simulink library "lib_Controller"  (R2017a)
settings: Solver=VariableStepAuto  StartTime=0.0  StopTime=10.0  RelTol=1e-3
undefined symbols (not defined in the file): cal, eng, ENGTRQ_MSMCH_Degraded_CP, ENGTRQ_MSMCH_ErrCritical_CP, ENGTRQ_MSMCH_LimpHome_CP
libraries: simulink x58, powerlib_meascontrol x3, lib_SystemDiag x1, EC2_libraries x1, lib_FuelManager x1, lib_TorqueDistribution x1
(part 3 of 3)

== system lib_Controller/Controller_with_Transmission_Manager1/HSC/Camaro Fault Detection/Signal Diagnostic/ESS Signal Diagnostic/Max charging voltage fault detect ==
  note: Note: When the ESS receives the energy from grid or regenerative braking,
      | the charging voltage to the inverter can not be bigger than 419V, otherwise the MCU will set to fault
  In1 : Inport
  " " : simulink/Logic and Bit Operations/Compare To Constant  relop=>  const=419  OutDataTypeStr=boolean
  Abs : Abs
  Compare To Zero : simulink/Logic and Bit Operations/Compare To Zero  relop=<  OutDataTypeStr=boolean
  Logical Operator : Logic  AllPortsSameDT=off  OutDataTypeStr=boolean
  Out1 : Outport
  wires:
  Abs/1 -> " "/1
  Logical Operator/1 -> Out1/1
  " "/1 -> Logical Operator/1
  In1/1 -> Compare To Zero/1, Abs/1
  Compare To Zero/1 -> Logical Operator/2

== system lib_Controller/Controller_with_Transmission_Manager1/HSC/Camaro Fault Detection/Signal Diagnostic/ESS Signal Diagnostic/Rolling Alive Counter Detection ==
  In1 : Inport
  Chart : Stateflow chart  TreatAsAtomicUnit=on
  Constant : Constant  Value=0.01
  Constant1 : Constant  Value=0.01
  Detect Change : simulink/Logic and Bit Operations/Detect Change  vinit=1  InputProcessing=Inherited  OutDataTypeStr=boolean
  Out1 : Outport
  wires:
  Constant1/1 -> Chart/3(tloop)
  In1/1 -> Detect Change/1
  Detect Change/1 -> Chart/1(PulseDetect)
  Chart/1(flag) -> Out1/1
  Constant/1 -> Chart/2(CycleTime)

== system lib_Controller/Controller_with_Transmission_Manager1/HSC/Camaro Fault Detection/Signal Diagnostic/ESS Signal Diagnostic/Validity Check ==
  In1 : Inport
  " Normal Operation" : simulink/Logic and Bit Operations/Compare To Constant  relop===  const=1  OutDataTypeStr=boolean
  Below Normal Operation : simulink/Logic and Bit Operations/Compare To Constant  relop===  const=0  OutDataTypeStr=boolean
  Logical Operator : Logic  Operator=OR  AllPortsSameDT=off  OutDataTypeStr=boolean
  Out1 : Outport
  wires:
  In1/1 -> Below Normal Operation/1, " Normal Operation"/1
  Below Normal Operation/1 -> Logical Operator/1
  " Normal Operation"/1 -> Logical Operator/2
  Logical Operator/1 -> Out1/1  "BMSgdf_SigValid"

== system lib_Controller/Controller_with_Transmission_Manager1/HSC/Camaro Fault Detection/Signal Diagnostic/Engine Signal Diagnostic/EngTempValidity_Check ==
  In1 : Inport
  Above Normal Operation : simulink/Logic and Bit Operations/Compare To Constant  relop===  const=3  OutDataTypeStr=boolean
  Logical Operator1 : Logic  Operator=NOT  AllPortsSameDT=off  OutDataTypeStr=boolean
  Out1 : Outport
  wires:
  Logical Operator1/1 -> Out1/1
  Above Normal Operation/1 -> Logical Operator1/1
  In1/1 -> Above Normal Operation/1

== system lib_Controller/Controller_with_Transmission_Manager1/HSC/Camaro Fault Detection/Signal Diagnostic/Engine Signal Diagnostic/Rolling Alive Counter Detection1 ==
  In1 : Inport
  Chart : Stateflow chart  TreatAsAtomicUnit=on
  Constant : Constant  Value=0.01
  Detect Change : simulink/Logic and Bit Operations/Detect Change  vinit=1  InputProcessing=Inherited  OutDataTypeStr=boolean
  Out1 : Outport
  wires:
  Constant/1 -> Chart/2(CycleTime)
  Chart/1(flag) -> Out1/1
  Detect Change/1 -> Chart/1(PulseDetect)
  In1/1 -> Detect Change/1

== system lib_Controller/Controller_with_Transmission_Manager1/HSC/Camaro Fault Detection/Signal Diagnostic/Transmission Signal Diagnostic/Rolling Alive Counter Detection ==
  In1 : Inport
  Chart : Stateflow chart  TreatAsAtomicUnit=on
  Constant : Constant  Value=0.01
  Detect Change : simulink/Logic and Bit Operations/Detect Change  vinit=1  InputProcessing=Inherited  OutDataTypeStr=boolean
  Out1 : Outport
  wires:
  Constant/1 -> Chart/2(CycleTime)
  Chart/1(flag) -> Out1/1
  Detect Change/1 -> Chart/1(PulseDetect)
  In1/1 -> Detect Change/1

== system lib_Controller/Controller_with_Transmission_Manager1/HSC/Camaro Fault Detection/Signal Diagnostic/Transmission Signal Diagnostic/Vehicle Direction Fault Detection ==
  LvrPosTrnsShft : Inport
  Speed : Inport  Port=2
  Compare To Constant : simulink/Logic and Bit Operations/Compare To Constant  relop===  const=4  OutDataTypeStr=boolean
  Compare To Constant1 : simulink/Logic and Bit Operations/Compare To Constant  relop=<  const=0  OutDataTypeStr=boolean
  Compare To Constant2 : simulink/Logic and Bit Operations/Compare To Constant  relop===  const=2  OutDataTypeStr=boolean
  Compare To Constant3 : simulink/Logic and Bit Operations/Compare To Constant  relop=>  const=0  OutDataTypeStr=boolean
  Logical Operator : Logic  AllPortsSameDT=off  OutDataTypeStr=boolean
  Logical Operator1 : Logic  AllPortsSameDT=off  OutDataTypeStr=boolean
  Logical Operator2 : Logic  Operator=OR  AllPortsSameDT=off  OutDataTypeStr=boolean
  Out1 : Outport
  wires:
  Logical Operator2/1 -> Out1/1
  Logical Operator/1 -> Logical Operator2/2
  Logical Operator1/1 -> Logical Operator2/1
  Compare To Constant3/1 -> Logical Operator1/2
  Compare To Constant2/1 -> Logical Operator1/1
  Compare To Constant/1 -> Logical Operator/1
  Compare To Constant1/1 -> Logical Operator/2
  Speed/1 -> Compare To Constant1/1, Compare To Constant3/1
  LvrPosTrnsShft/1 -> Compare To Constant/1, Compare To Constant2/1

== system lib_Controller/Controller_with_Transmission_Manager1/HSC/Driver_Requests/APP_BPP to DrvIntndAxlTrq2/Post Driver Intnded Axle Torque/Brake Command ==
  APP : Inport
  BPP : Inport  Port=2
  VehicleSpeed : Inport  Port=3
  1-D Lookup Table : Lookup_n-D  NumberOfTableDimensions=1  BreakpointsForDimension1=cal.Regen.BrakeAxleTrq.idx1_BrkPdlPos  Table=cal.Regen.BrakeAxleTrq.map  InternalRulePriority=Speed  RndMeth=Simplest  InputSameDT=on
  Compare To Constant : simulink/Logic and Bit Operations/Compare To Constant  relop=>=  const=cal.Regen.EnableSpeed  OutDataTypeStr=boolean
  Compare To Constant4 : simulink/Logic and Bit Operations/Compare To Constant  relop=<=  const=cal.Regen.EnableAPP  OutDataTypeStr=boolean
  Compare To Constant5 : simulink/Logic and Bit Operations/Compare To Constant  relop=>=  const=cal.Regen.DisableAPP  OutDataTypeStr=boolean
  Constant5 : Constant  Value=0
  Latch : Subsystem
  RegenCal : Gain  Gain=1.3
  Switch : Switch  Criteria=u2 > Threshold
  Terminator : Terminator
  BrkAxlTrq : Outport
  wires:
  VehicleSpeed/1 -> Compare To Constant/1
  1-D Lookup Table/1 -> RegenCal/1
  Switch/1 -> BrkAxlTrq/1
  APP/1 -> Compare To Constant5/1, Compare To Constant4/1
  BPP/1 -> 1-D Lookup Table/1
  Compare To Constant/1 -> Switch/2
  Constant5/1 -> Switch/3
  Compare To Constant5/1 -> Latch/2(Reset)
  Compare To Constant4/1 -> Latch/1(Input)
  Latch/1(Out1) -> Terminator/1
  RegenCal/1 -> Switch/1

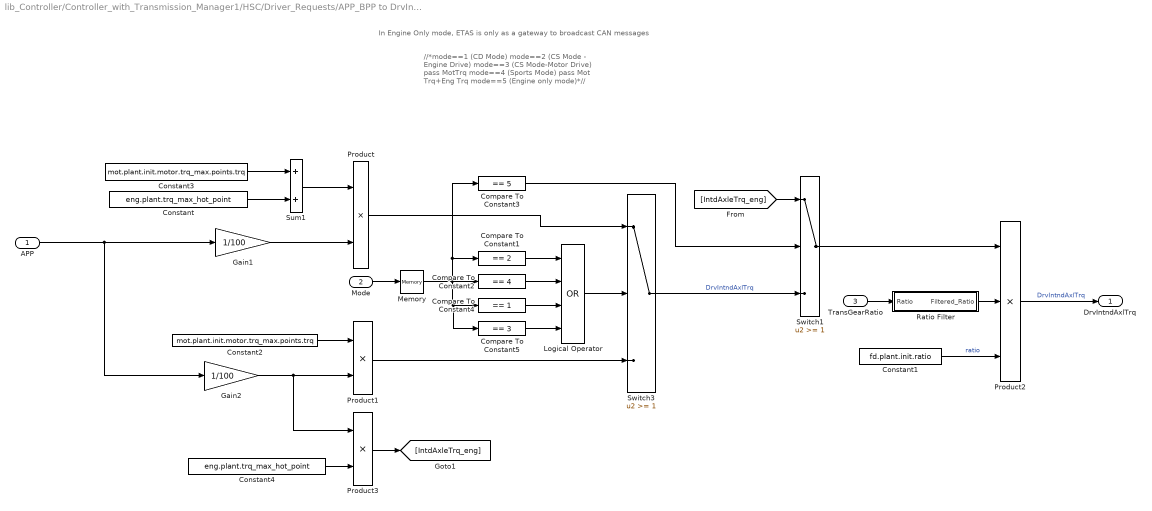
== system lib_Controller/Controller_with_Transmission_Manager1/HSC/Driver_Requests/APP_BPP to DrvIntndAxlTrq2/Post Driver Intnded Axle Torque/Driver Intended Axle Torque ==
  note: In Engine Only mode, ETAS is only as a gateway to broadcast CAN messages
  note: //*mode==1 (CD Mode)
      | mode==2 (CS Mode - Engine Drive)
      | mode==3 (CS Mode-Motor Drive) pass MotTrq
      | mode==4 (Sports Mode) pass Mot Trq+Eng Trq
      | mode==5 (Engine only mode)*//
  APP : Inport
  Mode : Inport  Port=2
  TransGearRatio : Inport  Port=3
  Compare To Constant1 : simulink/Logic and Bit Operations/Compare To Constant  relop===  const=2  OutDataTypeStr=boolean
  Compare To Constant2 : simulink/Logic and Bit Operations/Compare To Constant  relop===  const=4  OutDataTypeStr=boolean
  Compare To Constant3 : simulink/Logic and Bit Operations/Compare To Constant  relop===  const=5  OutDataTypeStr=boolean
  Compare To Constant4 : simulink/Logic and Bit Operations/Compare To Constant  relop===  const=1  OutDataTypeStr=boolean
  Compare To Constant5 : simulink/Logic and Bit Operations/Compare To Constant  relop===  const=3  OutDataTypeStr=boolean
  Constant : Constant  Value=eng.plant.trq_max_hot_point  VectorParams1D=off
  Constant1 : Constant  Value=fd.plant.init.ratio
  Constant2 : Constant  Value=mot.plant.init.motor.trq_max.points.trq  VectorParams1D=off
  Constant3 : Constant  Value=mot.plant.init.motor.trq_max.points.trq  VectorParams1D=off
  Constant4 : Constant  Value=eng.plant.trq_max_hot_point  VectorParams1D=off
  Gain1 : Gain  Gain=1/100
  Gain2 : Gain  Gain=1/100
  Logical Operator : Logic  Operator=OR  Inputs=4  AllPortsSameDT=off  OutDataTypeStr=boolean
  Memory : Memory
  Product : Product  RndMeth=Zero
  Product1 : Product  RndMeth=Zero
  Product2 : Product  Inputs=3  RndMeth=Zero
  Product3 : Product  RndMeth=Zero
  Ratio Filter : Subsystem
  Sum1 : Sum
  Switch1 : Switch  Threshold=1
  Switch3 : Switch  Threshold=1
  DrvIntndAxlTrq : Outport
  wires:
  Constant2/1 -> Product1/1
  Ratio Filter/1(Filtered_Ratio) -> Product2/2
  Gain2/1 -> Product1/2, Product3/1
  Product/1 -> Switch3/1
  Mode/1 -> Memory/1
  Constant1/1 -> Product2/3  "ratio"
  Product1/1 -> Switch3/3
  TransGearRatio/1 -> Ratio Filter/1(Ratio)
  Product2/1 -> DrvIntndAxlTrq/1  "DrvIntndAxlTrq"
  Gain1/1 -> Product/2
  Memory/1 -> Compare To Constant5/1, Compare To Constant4/1, Compare To Constant2/1, Compare To Constant3/1, Compare To Constant1/1
  Constant3/1 -> Sum1/1
  Compare To Constant1/1 -> Logical Operator/1
  Sum1/1 -> Product/1
  Compare To Constant2/1 -> Logical Operator/2
  Constant/1 -> Sum1/2
  Switch3/1 -> Switch1/3  "DrvIntndAxlTrq"
  Product3/1 -> [IntdAxleTrq_eng]
  Compare To Constant3/1 -> Switch1/2
  Constant4/1 -> Product3/2
  Logical Operator/1 -> Switch3/2
  [IntdAxleTrq_eng] -> Switch1/1
  Switch1/1 -> Product2/1
  APP/1 -> Gain2/1, Gain1/1
  Compare To Constant4/1 -> Logical Operator/3
  Compare To Constant5/1 -> Logical Operator/4

== system lib_Controller/Controller_with_Transmission_Manager1/HSC/Powertrain Manager/HV Manager/BMS_Manager/Fault Latch ==
  IsoFault : Inport
  Off Delay : powerlib_meascontrol/Logic/On Delay  DelayType=Off delay  delay=3  ic=0  Ts=0
      settings: SourceProductName=Simscape Power Systems
  IsoFaultLatched : Outport
  wires:
  IsoFault/1 -> Off Delay/1
  Off Delay/1 -> IsoFaultLatched/1

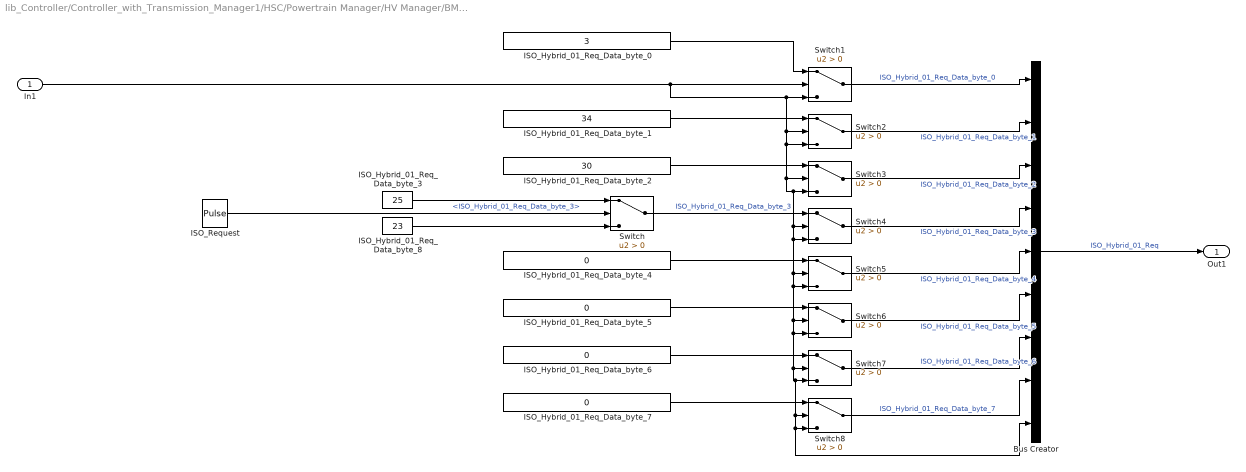
== system lib_Controller/Controller_with_Transmission_Manager1/HSC/Powertrain Manager/HV Manager/BMS_Manager/ISO_Hybrid_01_Req ==
  In1 : Inport
  Bus Creator : BusCreator  Inputs=9
  ISO_Hybrid_01_Req_Data_byte_0 : Constant  Value=3
  ISO_Hybrid_01_Req_Data_byte_1 : Constant  Value=34
  ISO_Hybrid_01_Req_Data_byte_2 : Constant  Value=30
  ISO_Hybrid_01_Req_Data_byte_3 : Constant  Value=25
  ISO_Hybrid_01_Req_Data_byte_{4..7} (4 alike) : Constant  Value=0
  ISO_Hybrid_01_Req_Data_byte_8 : Constant  Value=23
  ISO_Request : DiscretePulseGenerator  PulseType=Time based  Period=0.5  PulseWidth=50  SampleTime=-1
  Switch{,1..8} (9 alike) : Switch  Criteria=u2 > Threshold
  Out1 : Outport
  wires:
  Bus Creator/1 -> Out1/1  "ISO_Hybrid_01_Req"
  Switch6/1 -> Bus Creator/6  "ISO_Hybrid_01_Req_Data_byte_5"
  ISO_Hybrid_01_Req_Data_byte_8/1 -> Switch/3
  Switch5/1 -> Bus Creator/5  "ISO_Hybrid_01_Req_Data_byte_4"
  Switch3/1 -> Bus Creator/3  "ISO_Hybrid_01_Req_Data_byte_2"
  ISO_Hybrid_01_Req_Data_byte_3/1 -> Switch/1
  Switch1/1 -> Bus Creator/1  "ISO_Hybrid_01_Req_Data_byte_0"
  Switch7/1 -> Bus Creator/7  "ISO_Hybrid_01_Req_Data_byte_6"
  Switch2/1 -> Bus Creator/2  "ISO_Hybrid_01_Req_Data_byte_1"
  Switch8/1 -> Bus Creator/8  "ISO_Hybrid_01_Req_Data_byte_7"
  Switch4/1 -> Bus Creator/4  "ISO_Hybrid_01_Req_Data_byte_3"
  ISO_Hybrid_01_Req_Data_byte_0/1 -> Switch1/1
  In1/1 -> Switch2/2, Switch3/3, Switch4/3, Switch5/3, Switch6/3, Switch7/2, Switch7/3, Switch8/2, Bus Creator/9, Switch8/3, Switch6/2, Switch5/2, Switch4/2, Switch3/2, Switch2/3, Switch1/3, Switch1/2
  ISO_Hybrid_01_Req_Data_byte_1/1 -> Switch2/1
  ISO_Hybrid_01_Req_Data_byte_2/1 -> Switch3/1
  Switch/1 -> Switch4/1  "ISO_Hybrid_01_Req_Data_byte_3"
  ISO_Hybrid_01_Req_Data_byte_4/1 -> Switch5/1
  ISO_Hybrid_01_Req_Data_byte_5/1 -> Switch6/1
  ISO_Hybrid_01_Req_Data_byte_6/1 -> Switch7/1
  ISO_Hybrid_01_Req_Data_byte_7/1 -> Switch8/1
  ISO_Request/1 -> Switch/2  "<ISO_Hybrid_01_Req_Data_byte_3>"

== system lib_Controller/Controller_with_Transmission_Manager1/HSC/Powertrain Manager/HV Manager/BMS_Manager/Isolation Fault Calculation ==
  note: This block  allows to know which HV main
      | is having issues. HV POS 25, HV NEG 23.
  Sensors1 : Inport
  Bus Selector5 : BusSelector  OutputSignals=from_CAN.fromEBCAN.from_BMSAntrieb.ISO_Hybrid_01_Resp_Data.ISO_Hybrid_01_Resp_Data_byte_3,from_CAN.fromEBCAN.from_BMSAntrieb.ISO_Hybrid_01_Resp_Data.ISO_Hybrid_01_Resp_Data_byte_4,from_CAN.fromEBCAN.from_BMSAntrieb.ISO_Hybrid_01_Resp_Data.ISO_Hybrid_01_Resp_Data_byte_5
  Compare To Constant : simulink/Logic and Bit Operations/Compare To Constant  relop===  const=23  OutDataTypeStr=boolean
  Compare To Constant1 : simulink/Logic and Bit Operations/Compare To Constant  relop===  const=25  OutDataTypeStr=boolean
  HVnegativeISO : Constant  Value=0
  HVpositiveISO : Constant
  Logical Operator : Logic  Operator=OR  AllPortsSameDT=off  OutDataTypeStr=boolean
  POS or NEG HV MAIN : Switch  Criteria=u2 > Threshold  Threshold=24
  Resistance_Measurement : Subsystem
  Terminator8 : Terminator
  IsoFault : Outport
  wires:
  Resistance_Measurement/1(IsoFault) -> IsoFault/1
  POS or NEG HV MAIN/1 -> Terminator8/1
  Bus Selector5/2 -> Resistance_Measurement/1(In1)  "<ISO_Hybrid_01_Resp_Data_byte_4>"
  Bus Selector5/3 -> Resistance_Measurement/2(In2)  "<ISO_Hybrid_01_Resp_Data_byte_5>"
  Sensors1/1 -> Bus Selector5/1
  HVpositiveISO/1 -> POS or NEG HV MAIN/1
  Bus Selector5/1 -> POS or NEG HV MAIN/2, Compare To Constant1/1, Compare To Constant/1  "<ISO_Hybrid_01_Resp_Data_byte_3>"
  HVnegativeISO/1 -> POS or NEG HV MAIN/3
  Compare To Constant1/1 -> Logical Operator/1
  Compare To Constant/1 -> Logical Operator/2
  Logical Operator/1 -> Resistance_Measurement/Enable

== system lib_Controller/Controller_with_Transmission_Manager1/HSC/Powertrain Manager/HV Manager/DCDC Manager/Contactors status check ==
  note: Note: Contactors don't close when commanded
  BMS_Voltage : Inport
  BMS_LinkVoltage : Inport  Port=2
  BMS_HVILfault : Inport  Port=3
  " " : simulink/Logic and Bit Operations/Compare To Constant  relop=>  const=2  OutDataTypeStr=boolean
  Abs : Abs
  Logical Operator : Logic  Operator=OR  AllPortsSameDT=off  OutDataTypeStr=boolean
  Sum : Sum  Inputs=+-
  Out1 : Outport
  wires:
  BMS_Voltage/1 -> Sum/1
  Logical Operator/1 -> Out1/1  "BMS_contactorsFailed_Detected"
  Sum/1 -> Abs/1
  Abs/1 -> " "/1
  BMS_LinkVoltage/1 -> Sum/2
  BMS_HVILfault/1 -> Logical Operator/2
  " "/1 -> Logical Operator/1  "BMS_contactorsFailed_SigValid"

== system lib_Controller/Controller_with_Transmission_Manager1/HSC/Powertrain Manager/HV Manager/DCDC Manager/DCModeOverride ==
  In1 : Inport
  DCDCOVrrdSwitch : Constant  Value=0
  DCDCOVrrdVal : Constant  Value=0
  Switch : Switch  Criteria=u2 > Threshold
  Out1 : Outport
  wires:
  Switch/1 -> Out1/1  "DC_mode"
  In1/1 -> Switch/3
  DCDCOVrrdSwitch/1 -> Switch/2
  DCDCOVrrdVal/1 -> Switch/1

== system lib_Controller/Controller_with_Transmission_Manager1/HSC/Powertrain Manager/HV Manager/Inverter Manager/RequestOverride ==
  In1 : Inport
  ReqStateOVrRDSwitch : Constant  Value=0
  RequestedStateOvrRdValue : Constant
  Switch : Switch  Criteria=u2 > Threshold
  Out1 : Outport
  wires:
  Switch/1 -> Out1/1  "VCU_RequestedStateINV"
  In1/1 -> Switch/3
  ReqStateOVrRDSwitch/1 -> Switch/2
  RequestedStateOvrRdValue/1 -> Switch/1

== system lib_Controller/Controller_with_Transmission_Manager1/HSC/Camaro Fault Detection/Signal Diagnostic/ESS Signal Diagnostic/ESS SOC Validity Check/essSOCValidity_Check ==
  In1 : Inport
  Above Normal Operation : simulink/Logic and Bit Operations/Compare To Constant  relop===  const=3  OutDataTypeStr=boolean
  Below Normal Operation : simulink/Logic and Bit Operations/Compare To Constant  relop===  const=0  OutDataTypeStr=boolean
  Logical Operator : Logic  Operator=OR  AllPortsSameDT=off  OutDataTypeStr=boolean
  Logical Operator1 : Logic  Operator=NOT  AllPortsSameDT=off  OutDataTypeStr=boolean
  Out1 : Outport
  wires:
  In1/1 -> Above Normal Operation/1, Below Normal Operation/1
  Logical Operator/1 -> Logical Operator1/1
  Below Normal Operation/1 -> Logical Operator/1
  Above Normal Operation/1 -> Logical Operator/2
  Logical Operator1/1 -> Out1/1

== system lib_Controller/Controller_with_Transmission_Manager1/HSC/Camaro Fault Detection/Signal Diagnostic/ESS Signal Diagnostic/ESS Temp Validity Check/essTsignalValidity_Check ==
  In1 : Inport
  Above Normal Operation : simulink/Logic and Bit Operations/Compare To Constant  relop===  const=4  OutDataTypeStr=boolean
  Below Normal Operation : simulink/Logic and Bit Operations/Compare To Constant  relop===  const=0  OutDataTypeStr=boolean
  Logical Operator : Logic  Operator=OR  AllPortsSameDT=off  OutDataTypeStr=boolean
  Logical Operator1 : Logic  Operator=NOT  AllPortsSameDT=off  OutDataTypeStr=boolean
  Out1 : Outport
  wires:
  Logical Operator1/1 -> Out1/1
  Above Normal Operation/1 -> Logical Operator/2
  Below Normal Operation/1 -> Logical Operator/1
  Logical Operator/1 -> Logical Operator1/1
  In1/1 -> Below Normal Operation/1, Above Normal Operation/1

== system lib_Controller/Controller_with_Transmission_Manager1/HSC/Driver_Requests/APP_BPP to DrvIntndAxlTrq2/Post Driver Intnded Axle Torque/Brake Command/Latch ==
  Input : Inport
  Reset : Inport  Port=2
  Logical Operator1 : Logic  Operator=NOT  AllPortsSameDT=off  OutDataTypeStr=boolean
  Logical Operator2 : Logic  AllPortsSameDT=off  OutDataTypeStr=boolean
  Logical Operator3 : Logic  Operator=OR  AllPortsSameDT=off  OutDataTypeStr=boolean
  Memory1 : Memory
  Out1 : Outport
  wires:
  Logical Operator2/1 -> Logical Operator3/2
  Reset/1 -> Logical Operator1/1
  Memory1/1 -> Logical Operator2/2
  Logical Operator3/1 -> Out1/1, Memory1/1
  Logical Operator1/1 -> Logical Operator2/1
  Input/1 -> Logical Operator3/1

== system lib_Controller/Controller_with_Transmission_Manager1/HSC/Driver_Requests/APP_BPP to DrvIntndAxlTrq2/Post Driver Intnded Axle Torque/Driver Intended Axle Torque/Ratio Filter ==
  Ratio : Inport
  Abs : Abs
  Compare To Zero : simulink/Logic and Bit Operations/Compare To Zero  relop===  OutDataTypeStr=boolean
  Constant : Constant  Value=cal.Time.TrnsOvrllEstTrqRatioSwitch
  Mature_Delay : EC2_libraries/Mature_Delay
      settings: SourceProductName=The database C:\Users\vrajm\AppData\Roaming\MathWorks\MATLAB\R2017b\slblocks_master.db is locked, or a table in the database is locked. (database is locked)
  Memory1 : Memory  X0=1
  Switch1 : Switch  Threshold=1
  Switch2 : Switch  Threshold=1
  Filtered_Ratio : Outport
  wires:
  Ratio/1 -> Compare To Zero/1, Abs/1
  Compare To Zero/1 -> Mature_Delay/1, Switch2/2
  Abs/1 -> Switch1/1, Switch2/3
  Switch1/1 -> Switch2/1
  Constant/1 -> Mature_Delay/2
  Mature_Delay/1 -> Switch1/2
  Memory1/1 -> Switch1/3
  Switch2/1 -> Filtered_Ratio/1, Memory1/1  "gear_ratio"

== system lib_Controller/Controller_with_Transmission_Manager1/HSC/Powertrain Manager/HV Manager/BMS_Manager/Isolation Fault Calculation/Resistance_Measurement ==
  In1 : Inport
  In2 : Inport  Port=2
  Enable : EnablePort
  Add : Sum
  ISOfault : Constant
  ISOmultiplier : Constant  Value=256
  ISOnofault : Constant  Value=0
  Minimum Allowed Isolation Resistance : Switch  Criteria=u2 > Threshold  Threshold=500000
  Product : Product
  Product1 : Product
  Resistance Adjustment : Constant  Value=1000
  IsoFault : Outport
  wires:
  Minimum Allowed Isolation Resistance/1 -> IsoFault/1  "IsoFault"
  ISOnofault/1 -> Minimum Allowed Isolation Resistance/1
  Resistance Adjustment/1 -> Product1/2
  Product1/1 -> Minimum Allowed Isolation Resistance/2
  ISOfault/1 -> Minimum Allowed Isolation Resistance/3
  Add/1 -> Product1/1
  Product/1 -> Add/1
  In2/1 -> Add/2
  In1/1 -> Product/1
  ISOmultiplier/1 -> Product/2

== stateflow chart lib_Controller/Controller_with_Transmission_Manager1/HSC/Camaro Fault Detection/Component Diagnostic/Driver Input Diagnostic/Driver_Input_Diag ==
  state Driver_Input_Offline
    en: Driver_Input_Status=0;
  state Driver_Input_Online
    en: Driver_Input_Status=1;
  (default) -> Driver_Input_Offline
  Driver_Input_Online -> Driver_Input_Offline : [~APP_Valid|| ~Drv_BPP_SigValid||~KeyPos||~PRNDL||BrakeFail]
  Driver_Input_Offline -> Driver_Input_Online : [APP_Valid&&Drv_BPP_SigValid&&KeyPos&&PRNDL&&BrakeFail==0]
  data: APP_Valid input; Drv_BPP_SigValid input; KeyPos input; Driver_Input_Status output; PRNDL input; BrakeFail input

== stateflow chart lib_Controller/Controller_with_Transmission_Manager1/HSC/Camaro Fault Detection/Component Diagnostic/ESS Component Diagnostic/BMS_CompDiag1 ==
  state BMS_Offline
    en: BMS_Status=0;
  state BMS_Online
    en:BMS_Status=2;
  state BMS_Limited
    en: BMS_Status=1;
  BMS_Offline -> BMS_Online [order 1] : [BMS_RollingAliveActive_SigValid&&BMS_contactorsFailed_SigValid&&...
      | BMS_essTemp_SigValid&&ClearFault&&BMS_essSOC_0_1_SigValid&&...
      | ess_GroundFault&&essCur_A_SigValid]
  (default) -> BMS_Offline
  BMS_Online -> BMS_Offline [order 2] : [~BMS_RollingAliveActive_SigValid||...
      | ~BMS_contactorsFailed_SigValid||~BMS_essSOC_0_1_SigValid|| ...
      | ~ess_GroundFault]
  BMS_Limited -> BMS_Offline [order 2] : [~BMS_RollingAliveActive_SigValid||...
      | ~BMS_contactorsFailed_SigValid]
  BMS_Offline -> BMS_Limited [order 2] : [BMS_RollingAliveActive_SigValid &&...
      | BMS_contactorsFailed_SigValid && ~BMS_essTemp_SigValid||...
      |  ~BMS_essSOC_0_1_SigValid]
  BMS_Limited -> BMS_Online [order 1] : [BMS_essTemp_SigValid||...
      | ClearFault||BMS_essSOC_0_1_SigValid]
  BMS_Online -> BMS_Limited [order 1] : [~BMS_essTemp_SigValid||...
      |  ~BMS_essSOC_0_1_SigValid]
  data: BMS_RollingAliveActive_SigValid input; BMS_contactorsFailed_SigValid input; BMS_essTemp_SigValid input; BMS_Status output; BMS_essSOC_0_1_SigValid input; essCur_A_SigValid input; ess_GroundFault input; ClearFault input

== stateflow chart lib_Controller/Controller_with_Transmission_Manager1/HSC/Camaro Fault Detection/Component Diagnostic/Engine Component Diagnostic/ECM_CompDiag ==
  state ECM_Offline
    en: ECM_Status=0;
  state ECM_Online
    en:ECM_Status=2;
  state ECM_Limited
    en: ECM_Status=1;
  ECM_Online -> ECM_Offline [order 2] : [~ECM_RollingAliveActive||~engTrqCmdRecvd_SigValid||...
      | ~Engine_Speed_rpm_SigValid||Eng_TempRange_123==3||Eng_Torq_Msmch==1||ClearFault==0]
  (default) -> ECM_Offline
  ECM_Offline -> ECM_Online [order 1] : [ECM_RollingAliveActive&&engTrqCmdRecvd_SigValid &&...
      | Engine_Speed_rpm_SigValid&&ClearFault&&Eng_TempRange_123==1&&Eng_Torq_Msmch==0&&ClearFault]
  ECM_Limited -> ECM_Offline [order 2] : [~ECM_RollingAliveActive||~engTrqCmdRecvd_SigValid||~Engine_Speed_rpm_SigValid|| Eng_TempRange_123==3||Eng_Torq_Msmch==1]
  ECM_Offline -> ECM_Limited [order 2] : [ECM_RollingAliveActive...
      | &&engTrqCmdRecvd_SigValid &&Engine_Speed_rpm_SigValid...
      | &&Eng_Torq_Msmch==0&&[Eng_TempRange_123==2 ]]
  ECM_Online -> ECM_Limited [order 1] : [ECM_RollingAliveActive...
      | &&engTrqCmdRecvd_SigValid &&Engine_Speed_rpm_SigValid...
      | &&Eng_Torq_Msmch==0&&(Eng_TempRange_123==2 )]
  ECM_Limited -> ECM_Online [order 1] : [Eng_TempRange_123==1&&Eng_Torq_Msmch==0]
  data: ECM_RollingAliveActive input; engTrqCmdRecvd_SigValid input; Eng_Torq_Msmch input; Engine_Speed_rpm_SigValid input; Eng_TempRange_123 input; ECM_Status output; ClearFault input

== stateflow chart lib_Controller/Controller_with_Transmission_Manager1/HSC/Camaro Fault Detection/Component Diagnostic/Engine Component Diagnostic/Eng_Torq_MsmchLevel ==
  state Normal_Torque
    en: Eng_Torq_MsmchLevel==1
  state Creep_Torq_Allowed
    en: Eng_Torq_MsmchLvel==3
  state AboveMax
    en: Eng_Torq_MsmchLevel==4
  state Max_power_limited
    en: Eng_Torq_MsmchLvel==2
  (default) -> Normal_Torque
  AboveMax -> Normal_Torque [order 2] : [SignalValue<ENGTRQ_MSMCH_Degraded_CP]
  Creep_Torq_Allowed -> AboveMax [order 2] : [SignalValue>ENGTRQ_MSMCH_ErrCritical_CP]
  Max_power_limited -> Normal_Torque [order 1] : [SignalValue<ENGTRQ_MSMCH_Degraded_CP]
  Normal_Torque -> Max_power_limited [order 1] : [SignalValue>ENGTRQ_MSMCH_Degraded_CP&&...
      | SignalValue<ENGTRQ_MSMCH_LimpHome_CP]
  Normal_Torque -> AboveMax [order 2] : [SignalValue>ENGTRQ_MSMCH_ErrCritical_CP]
  AboveMax -> Creep_Torq_Allowed [order 1] : [SignalValue>ENGTRQ_MSMCH_LimpHome_CP&&SignalValue<ENGTRQ_MSMCH_ErrCritical_CP]
  Creep_Torq_Allowed -> Max_power_limited [order 1] : [SignalValue<ENGTRQ_MSMCH_LimpHome_CP&&SignalValue>ENGTRQ_MSMCH_Degraded_CP]
  Max_power_limited -> Creep_Torq_Allowed [order 2] : [SignalValue>ENGTRQ_MSMCH_LimpHome_CP&&SignalValue<ENGTRQ_MSMCH_ErrCritical_CP]
  data: SignalValue input; ENGTRQ_MSMCH_Degraded_CP parameter; ENGTRQ_MSMCH_LimpHome_CP parameter; Eng_Torq_MsmchLevel output; ENGTRQ_MSMCH_ErrCritical_CP parameter

== stateflow chart lib_Controller/Controller_with_Transmission_Manager1/HSC/Camaro Fault Detection/Signal Diagnostic/Driver Signal Diagnostic/AccPedalValidity ==
  state SignalHigh
    en: signalValid=0;
  state SignalInRange
  state SignalLow
    en:signalValid=0;
  SignalHigh -> SignalInRange : [signalValue<=100]
  SignalInRange -> SignalHigh [order 1] : [signalValue>102]
  SignalInRange -> SignalInRange [order 3] : [clearFaults==1]
      | {signalValid=1;}
  (default) -> SignalInRange : {signalValid=1;}
  SignalLow -> SignalInRange : [signalValue>0]
  SignalInRange -> SignalLow [order 2] : [signalValue<-0.5]
  data: clearFaults input; signalValue input; signalValid output

== stateflow chart lib_Controller/Controller_with_Transmission_Manager1/HSC/Camaro Fault Detection/Signal Diagnostic/Driver Signal Diagnostic/AccPedalValidity1 ==
  state SignalHigh
    en: signalValid=0;
  state SignalInRange
  state SignalLow
    en:signalValid=0;
  SignalHigh -> SignalInRange : [signalValue<=100]
  SignalInRange -> SignalHigh [order 1] : [signalValue>102]
  SignalInRange -> SignalInRange [order 3] : [clearFaults==1]
      | {signalValid=1;}
  (default) -> SignalInRange : {signalValid=1;}
  SignalLow -> SignalInRange : [signalValue>0]
  SignalInRange -> SignalLow [order 2] : [signalValue<-0.5]
  data: clearFaults input; signalValue input; signalValid output

== stateflow chart lib_Controller/Controller_with_Transmission_Manager1/HSC/Camaro Fault Detection/Signal Diagnostic/Driver Signal Diagnostic/BrakeFailureDetection/Chart ==
  state No_Fault
    en:
    DecelFail=0;
  state Detection_State
    en:
    Detection_state=1;
  state No_Fault1
    en:
    DecelFail=0;
  state Detection_State1
    en:
    Detection_state=2;
  state No_Fault2
    en:
    DecelFail=0;
  state Detection_State2
    en:
    Detection_state=3;
    du:
    DecelFail=1;
  (default) -> (junction 3)
  (junction 3) -> No_Fault [order 2]
  (junction 3) -> Detection_State [order 1] : [VehSpeed>0]
  Detection_State -> (junction 8)
  (junction 8) -> No_Fault1 [order 2]
  (junction 8) -> Detection_State1 [order 1] : [BPP>0]
  Detection_State1 -> (junction 15)
  (junction 15) -> No_Fault2 [order 2]
  (junction 15) -> Detection_State2 [order 1] : [Incre||Unchange]
  data: BPP input; VehSpeed input; Incre input; Unchange input; DecelFail output; Detection_state local

== stateflow chart lib_Controller/Controller_with_Transmission_Manager1/HSC/Camaro Fault Detection/Signal Diagnostic/ESS Signal Diagnostic/ESS SOC Validity Check/essSOC_0_1Range ==
  state aboveMax
    en: essSOCRange=3;
  state NormalRange
    en: essSOCRange=2;
  state LowRange
    en:essSOCRange=1;
  state BelowNormal
    en: essSOCRange=0;
  aboveMax -> NormalRange : [signalValue<0.95]
  NormalRange -> aboveMax [order 1] : [signalValue>=0.95]
  NormalRange -> NormalRange [order 3] : [clearFaults==1]
      | {essSOCRange=2;}
  (default) -> NormalRange
  LowRange -> NormalRange [order 1] : [signalValue>0.3]
  NormalRange -> LowRange [order 2] : [signalValue<=0.3&&signalValue>0.15]
  LowRange -> BelowNormal [order 2] : [signalValue<=0.15]
  BelowNormal -> LowRange : [signalValue>0.15]
  data: clearFaults input; signalValue input; data local; essSOCRange output

== stateflow chart lib_Controller/Controller_with_Transmission_Manager1/HSC/Camaro Fault Detection/Signal Diagnostic/ESS Signal Diagnostic/ESS Temp Validity Check/essTsignalRange ==
  state AboveMax
    en: essTempRange=4;
  state HighRange
    en: essTempRange=3;
  state NormalRange
    en: essTempRange=2;
  state LowRange
    en:essTempRange=1;
  state BelowNormal
    en: essTempRange=0;
  HighRange -> AboveMax [order 2] : [signalValue>55]
  AboveMax -> HighRange : [signalValue<55]
  HighRange -> NormalRange [order 1] : [signalValue<=30]
  NormalRange -> HighRange [order 1] : [signalValue>32]
  NormalRange -> NormalRange [order 3] : [clearFaults==1]
      | {essTempRange=2;}
  (default) -> NormalRange
  LowRange -> NormalRange [order 1] : [signalValue>=30]
  NormalRange -> LowRange [order 2] : [signalValue<0 ]
  LowRange -> BelowNormal [order 2] : [signalValue<-28]
  BelowNormal -> LowRange : [signalValue>28]
  data: clearFaults input; signalValue input; essTempRange output; data local

== stateflow chart lib_Controller/Controller_with_Transmission_Manager1/HSC/Camaro Fault Detection/Signal Diagnostic/ESS Signal Diagnostic/Rolling Alive Counter Detection/Chart ==
  state Off
    en:flag=0;
  state Alive
    en:flag=1;
  state Dead
    en:flag=0;
  Alive -> Alive [order 1] : after(CycleTime-tloop,sec)
      | [PulseDetect==1]
  (default) -> Off
  Off -> Alive : [PulseDetect==1]
  Alive -> Dead [order 2] : after(CycleTime,sec)
  data: PulseDetect input; CycleTime input; flag output; tloop input

== stateflow chart lib_Controller/Controller_with_Transmission_Manager1/HSC/Camaro Fault Detection/Signal Diagnostic/Engine Signal Diagnostic/Rolling Alive Counter Detection1/Chart ==
  state Off
    en:flag=0;
  state Alive
    en:flag=1;
  state Dead
    en:flag=0;
  Alive -> Alive [order 1] : after(CycleTime-tloop,sec)
      | [PulseDetect==1]
  (default) -> Off
  Off -> Alive : [PulseDetect==1]
  Alive -> Dead [order 2] : after(CycleTime,sec)
  data: PulseDetect input; CycleTime input; flag output; tloop parameter

== stateflow chart lib_Controller/Controller_with_Transmission_Manager1/HSC/Camaro Fault Detection/Signal Diagnostic/Transmission Signal Diagnostic/Rolling Alive Counter Detection/Chart ==
  state Off
    en:flag=0;
  state Alive
    en:flag=1;
  state Dead
    en:flag=0;
  Alive -> Alive [order 1] : after(CycleTime-tloop,sec)
      | [PulseDetect==1]
  (default) -> Off
  Off -> Alive : [PulseDetect==1]
  Alive -> Dead [order 2] : after(CycleTime,sec)
  data: PulseDetect input; CycleTime input; flag output; tloop parameter

== stateflow chart lib_Controller/Controller_with_Transmission_Manager1/HSC/Powertrain Manager/HV Manager/BMS_Manager/ESS_Manager ==
  state Fault_light_OFF
    entry: GFD_Light=0;
  state Ground_Fault
    entry:
    HV_State=-7;
    GFD_Light=1
  state Voltage_Fault
  state HVIL_Fault
    entry: MO_BMS_Sollmodus=0;
    HV_State=-8
  state HV_Startup
    state Drive_State
      entry:  HV_State=1;
      T_15=1;
      T_30=1;
      HVDischarge=0;
    state Contactor
      entry:
      T_30C=1;
    state Clear_Faults
      entry:
      Diag_Rq_Fktnl_Data_OBD_byte_0 =1;
      Diag_Rq_Fktnl_Data_OBD_byte_1=4;
      Diag_Rq_Fktnl_Data_OBD_byte_2=0;
      Diag_Rq_Fktnl_Data_OBD_byte_3=0;
      Diag_Rq_Fktnl_Data_OBD_byte_4=0;
      Diag_Rq_Fktnl_Data_OBD_byte_5=0;
      Diag_Rq_Fktnl_Data_OBD_byte_6=0;
      Diag_Rq_Fktnl_Data_OBD_byte_7=0;
      HV_State=2;
    state Charge_Wake
      entry: chga_wake=1;
      HV_State=3;
    state Drive_Wake
      entry: veh_wake=1;
      HV_State=8;
    state BMS_Enable_Charge
      entry: MO_BMS_Sollmodus=0;
      % T_15=1;
      % T_30C=1;
      HV_State=4;
    state BMS_Enable_Drive
      entry: MO_BMS_Sollmodus=0;
      HV_State=9;
    state Power_Contactors_Drive
      en: MO_BMS_Sollmodus=0;
      HV_State=10;
    state Power_Contactors_Charge
      en: MO_BMS_Sollmodus=0;
      %T_30C=1;
      HV_State=5;
    state Close_Contactors_Drive
      entry:
      MO_BMS_Sollmodus=1;
      HV_State=11;
    state Close_Contactors_Charge
      entry:
      MO_BMS_Sollmodus=1;
      HV_State=6;
    state Time_delay
    state Ready_to_Charge
      entry: ReadyToCharge=1;
      ISO_Hybrid_01_Req = 1;
      HV_State=7;
    state Ready_to_Drive
      entry: ReadyToDrive=1;
      ISO_Hybrid_01_Req = 1;
      HV_State=12;
    (default) -> Contactor
    Contactor -> Drive_State : after(0.25,sec)
    Drive_State -> Clear_Faults : after(0.1,sec)
    Clear_Faults -> Charge_Wake [order 1] : [plugged]
    Clear_Faults -> Drive_Wake [order 2] : %after(0.1,sec)
    Drive_Wake -> BMS_Enable_Drive : [BMS_Fehler_Pilot==0 ]
    Charge_Wake -> BMS_Enable_Charge : [BMS_Fehler_Pilot==0 ]
    BMS_Enable_Charge -> Power_Contactors_Charge : [BMS_Init_abgeschlossen]
    BMS_Enable_Drive -> Power_Contactors_Drive : [BMS_Init_abgeschlossen]
    Power_Contactors_Drive -> Close_Contactors_Drive : [closeMaincReq]
    Power_Contactors_Charge -> Close_Contactors_Charge : [closeMaincReq]
    Close_Contactors_Charge -> Time_delay : [BMS_Fehler_HS_offen==0&&(BMS_IstModus==4||BMS_IstModus==1)]
    Close_Contactors_Drive -> Ready_to_Drive : [BMS_Fehler_HS_offen==0&&BMS_IstModus==1]
    Time_delay -> Ready_to_Charge : after(1,sec)
    Ready_to_Drive -> Ready_to_Charge : [plugged]
    Ready_to_Charge -> Ready_to_Drive : [plugged==0]
  note: // Rev 2_14_2017
      | Added plugged to Off-On transition
      | Added EnableInverter to charge path
      | Changed IstModus to 1 at the end of charge path
      |
      | Create HV On Request block to request charging when vehicle is off
  state HV_Shudown
    state Open_Contactors
      entry: MO_BMS_Sollmodus=0;
      HV_State=-1;
      ISO_Hybrid_01_Req = 0;
    state ShutDown_T30C
      entry: T_30C=0;
    state Discharge_Bus
      entry: HVDischarge=1;
      HV_State=-2;
    state Disable_BCM_1
      entry: T_15=0;
      HVDischarge=0;
      HV_State=-3;
    state Disable_BCM_2
      entry: T_30=0;
      HVDischarge=0;
      HV_State=-4;
    state Send_BCM_to_Sleep
      en: MO_SleepAckn =1;
      T_15=0;
      T_30=0;
      HV_State=-5;
    state Shutdown_Complete
      entry: Shutdown_Complete=1;
      HV_State=-6;
    (default) -> Open_Contactors
    Open_Contactors -> ShutDown_T30C : after(2,sec)
    ShutDown_T30C -> Discharge_Bus : [BMS_IstModus==5]
    Discharge_Bus -> Disable_BCM_1 : [BMS_Spannung_ZwKr<30]
    Disable_BCM_1 -> Disable_BCM_2 : [BMS_IstStrom<0.02]
    Disable_BCM_2 -> Send_BCM_to_Sleep
    Send_BCM_to_Sleep -> Shutdown_Complete : [BMS_SleepInd]
  note: //Rev 8_21_2017
      | //Removed all engine related conditions
      | //Removed EngRunATV
  Voltage_Fault -> HV_Shudown [order 1] : after(0.5, sec)
  Ground_Fault -> Fault_light_OFF : [(ISOfault==0&&KeyPos==1)||(ISOfault==0&&KeyPos==0&&plugged==1)]
  HV_Shudown -> Ground_Fault [order 2] : [ISOfault==1]
  Fault_light_OFF -> HV_Shudown
  HV_Startup -> Ground_Fault [order 3] : [ISOfault==1]
  HV_Startup -> HVIL_Fault [order 4] : [BMS_Fehler_Pilot]
  HVIL_Fault -> HV_Shudown : [BMS_Fehler_Pilot==0]
  HV_Startup -> Voltage_Fault [order 2] : after(5,sec)
      | [BMS_Spannung_ZwKr<50&&EngRunAtv]
  Voltage_Fault -> HV_Startup [order 2] : after(1,sec)
  (default) -> HV_Shudown
  HV_Shudown -> HV_Startup [order 1] : [HV_req==1||plugged||EngRunAtv]
  HV_Startup -> HV_Shudown [order 1] : [closeMaincReq==0&&plugged==0]
      | {ReadyToDrive = 0;
      | ReadyToCharge = 0;}
  data: data local; ISOfault input; plugged input; BMS_Fehler_HS_offen input; BMS_Fehler_Pilot input; BMS_Init_abgeschlossen input; BMS_IstModus input; BMS_IstSpannung input; BMS_IstStrom input; BMS_SleepInd input; Diag_Rq_Fktnl_Data_OBD_byte_0 output; Diag_Rq_Fktnl_Data_OBD_byte_1 output; Diag_Rq_Fktnl_Data_OBD_byte_2 output; Diag_Rq_Fktnl_Data_OBD_byte_3 output; Diag_Rq_Fktnl_Data_OBD_byte_4 output; Diag_Rq_Fktnl_Data_OBD_byte_5 output; Diag_Rq_Fktnl_Data_OBD_byte_6 output; Diag_Rq_Fktnl_Data_OBD_byte_7 output; ISO_Hybrid_01_Req output; MO_SleepAckn output; MO_BMS_Sollmodus output; T_15 output; T_30 output; T_30C output; veh_wake output; chga_wake output; HVDischarge output; HV_State output; ReadyToDrive output; ReadyToCharge output; Shutdown_Complete output; HV_req input boolean; BMS_Spannung_ZwKr input; NMH_BMS_Car_WakeUp input; NMH_Normal_Mode_1 input; NMH_BMS_Normal_Mode_2 input; NMH_BMS_Start_1 input; NMH_BMS_Start_2 input; timer local; KeyPos input; GFD_Light output; EngRunAtv input; closeMaincReq input boolean

== stateflow chart lib_Controller/Controller_with_Transmission_Manager1/HSC/Powertrain Manager/HV Manager/DCDC Manager/DCDCManager ==
  state DCDC_Initialization
    state Initialization
      entry: DCDC_State = 1;
    state Power_On
      entry: DCmode = 1;
      DCDC_State = 2;
      VoltageHV = 0;
      VoltageLV =14;
      CurrentHV = 20;
      CurrentLV = 173;
    (default) -> Initialization
    Initialization -> Power_On : [ContactorsFailed == 0]
  state Delay
  state DCDC_Off
    entry: DCDC_State = 4;
    DCmode = 0;
  (default) -> DCDC_Initialization
  Delay -> DCDC_Initialization : after(5,sec)
  DCDC_Initialization -> DCDC_Off : [INV_state == 14 || ...
      | ContactorsFailed == 1|| ...
      | mode == 7]
  DCDC_Off -> Delay : [(INV_state == 3 || INV_state == 8) && ...
      | ContactorsFailed == 0&&...
      |  (powerMode ==1|| powerMode == 2 || powerMode == 3)]
  data: ContactorsFailed input; DCmode output; VoltageHV output; CurrentHV output; VoltageLV output; CurrentLV output; INV_state input; DCDC_State output; mode input; powerMode input

== stateflow chart lib_Controller/Controller_with_Transmission_Manager1/HSC/Powertrain Manager/HV Manager/Inverter Manager/MCU_Manager  ==
  state MCU_Initialization
    state MCU_Request_Standby
      en:
      MCU_State = 1;
      RequestedStateINV = 3;
      CAN_Activation = 1;
    state Power_Off_INVCON
      entry:
      MCU_State = 0;
      INVCON_Power =0;
    state Power_On_INVCON
      en:MCU_State = 2;
      INVCON_Power =1;
    state HV_CAN_Actuation_Fault
      en:
      MCU_State = -1;
      CAN_Activation = 0;
    state INVCON_Power_Fault
      en:
      MCU_State = -2;
      INVCON_Power =0;
      CAN_Activation = 0;
    Power_Off_INVCON -> (junction 18) : {Timer=0;}
    (junction 18) -> MCU_Request_Standby [order 1] : [HVCAN_State]
    (default) -> Power_Off_INVCON
    HV_CAN_Actuation_Fault -> (junction 18) : [HVCAN_State]
    (junction 18) -> HV_CAN_Actuation_Fault [order 2] : after(3,sec)
    INVCON_Power_Fault -> (junction 18) : [~INVCON_Power_Feedback]
    MCU_Request_Standby -> Power_On_INVCON : after(5,sec)
    Power_On_INVCON -> INVCON_Power_Fault : after(5,sec)
        | [INV_State ~= 3]
  state MCU_ChargeMode
    state MCU_Ready
      en:
      MCU_State = 7;
    state MCU_Off
      en:
      MCU_State = 8;
      RequestedStateINV = 3;
    (default) -> MCU_ChargeMode.MCU_Ready
    MCU_ChargeMode.MCU_Ready -> MCU_ChargeMode.MCU_Off : [~ReadyToCharge]
  state MCU_TorqueMode
    state MCU_Enable
      en:MCU_State = 4;
      RequestedStateINV = 8;
      during: Timer = Timer + 1;
    state MCU_Ready
      en:
      MCU_State = 3;
    state MCU_Running
      en:
      MCU_State =5;
    state TorqueCommand_Reject_Fault
      en:
      MCU_State = -3;
    state MCU_Stop
      en:
      MCU_State = 6;
      RequestedStateINV = 3;
    (default) -> MCU_TorqueMode.MCU_Ready
    MCU_Enable -> (junction 35)
    (junction 35) -> MCU_Running [order 1] : [INV_State == 8]
    MCU_TorqueMode.MCU_Ready -> MCU_Enable : [EnableInverter]
        | {Timer = 0;}
    (junction 35) -> TorqueCommand_Reject_Fault [order 2] : after(5,sec)
    MCU_Running -> MCU_Stop : [~ReadyToDrive]
  state MCU_Shutdown
    state MCU_Off
      en:
      MCU_State = 10;
      RequestedStateINV = 0;
      during: Timer=Timer+1;
    state MCU_RdyForShtDwn
      en:
      MCU_State = 9;
    state MCU_Shtdwn_Cmplt
      en:
      MCU_State = 11;
      INVCON_Power =0;
      CAN_Activation = 0;
    state Motor_Isolate
      en:
      MCU_State = -5;
      INVCON_Power = 0;
      Motor_Torque_Command = 0;
    state ShutdownReq_Reject_Fault
      en:
      MCU_State = -4;
    (default) -> MCU_RdyForShtDwn
    MCU_RdyForShtDwn -> MCU_Shutdown.MCU_Off : [~EnableInverter]
        | {Timer = 0;}
    MCU_Shutdown.MCU_Off -> (junction 55)
    (junction 55) -> MCU_Shtdwn_Cmplt [order 2] : [INV_State == 0]
    (junction 55) -> ShutdownReq_Reject_Fault [order 1] : after(5,sec)
        | [INV_State == 14]
    ShutdownReq_Reject_Fault -> Motor_Isolate : after(3,sec)
  (default) -> MCU_Initialization
  MCU_Shutdown -> MCU_Initialization : [EnableInverter]
  MCU_TorqueMode -> MCU_Initialization [order 1] : [INV_State == 14]
  MCU_Initialization -> MCU_TorqueMode [order 2] : [INV_State == 3 &&...
      |  INVCON_Power_Feedback && ReadyToDrive]
  MCU_Initialization -> MCU_ChargeMode [order 1] : [INV_State == 3 &&...
      |  INVCON_Power_Feedback && ReadyToCharge]
  MCU_ChargeMode -> MCU_Initialization [order 2] : [INV_State == 14]
  MCU_TorqueMode -> MCU_Shutdown [order 2] : [INV_State == 3 && ~ReadyToDrive]
  MCU_ChargeMode -> MCU_Shutdown [order 1] : [INV_State == 3 && ~ReadyToCharge]
  data: ReadyToDrive input boolean; ReadyToCharge input; HVCAN_State input boolean; INVCON_Power_Feedback input; INV_State input; INV_CurrentHV input; Timer local double; MCU_State output; EnableInverter input boolean; ShutdownCurrent input; Motor_Torque_Command output; INVCON_Power output double; RequestedStateINV output; CAN_Activation output

== stateflow chart lib_Controller/Controller_with_Transmission_Manager1/HSC/Camaro Fault Detection/Component Diagnostic/Transmission Component Diagnostic/TCM_CompDia ==
  state TCM_Offline
    en: TCM_Status=0;
  state TCM_Limited [commented out]
    en: TCM_Status=1;
  state TCM_Online
    en: TCM_Status=2;
  (default) -> TCM_Offline
  TCM_Online -> TCM_Offline : [~TCMRollingAliveActive_SigValid||...
      | ~LvrPosTrnsShft_SigValid||...
      | ~TransEstGear_SigValid||...
      | ~LockupCmd_SigValid||VehDirFault]
  TCM_Offline -> TCM_Online : [TCMRollingAliveActive_SigValid&&...
      | LvrPosTrnsShft_SigValid&&TransEstGear_SigValid&&...
      | LockupCmd_SigValid&&VehDirFault==0]
  TCM_Online -> TCM_Limited [commented out]
  TCM_Limited -> TCM_Online [commented out]
  data: TCM_Status output; TCMRollingAliveActive_SigValid input; LvrPosTrnsShft_SigValid input; TransEstGear_SigValid input; LockupCmd_SigValid input; VehDirFault input

== stateflow chart lib_Controller/Controller_with_Transmission_Manager1/HSC/Camaro Fault Detection/Input Conversions/TCM_Conversions/TCM_RollinAliveCounter/Rolling Alive Counter1 ==
  state RollingAliveCounter
    state Count1
      en: RollingAliveCnt=0;
    state Count2
      en: RollingAliveCnt=1;
    state Count3
      en: RollingAliveCnt=2;
    state Count4
      en: RollingAliveCnt=3;
    (default) -> Count1
    Count4 -> Count1 : after(0.01,sec)
    Count1 -> Count2 : after(0.01,sec)
    Count2 -> Count3 : after(0.01,sec)
    Count3 -> Count4 : after(0.01,sec)
  data: RollingAliveCnt output double

== stateflow chart lib_Controller/Controller_with_Transmission_Manager1/HSC/Camaro Fault Detection/Signal Diagnostic/Engine Signal Diagnostic/Engine_Temp[DegC] ==
  state AboveMax
    en: EngTempRange=3;
  state HighRange
    en: EngTempRange=2;
  state NormalRange
    en: EngTempRange=1;
  HighRange -> AboveMax [order 2] : [Engine_Temp_DegC>120]
  AboveMax -> HighRange : [Engine_Temp_DegC<120]
  NormalRange -> HighRange [order 1] : [Engine_Temp_DegC>100&&Engine_Temp_DegC<120]
  HighRange -> NormalRange [order 1] : [Engine_Temp_DegC<=100]
  NormalRange -> NormalRange [order 2] : [clearFaults==1]
      | {EngTempRange=1;}
  (default) -> NormalRange
  data: clearFaults input; Engine_Temp_DegC input; EngTempRange output; data local
